simulink model "GlidePathControl_GlideSlopeAngle"  (R2018b)
settings: Solver=VariableStepAuto  StartTime=0.0  StopTime=30  RelTol=1e-3
libraries: simulink x1
settings Model: Creator=cdjsd  LastModifiedBy=cdjsd

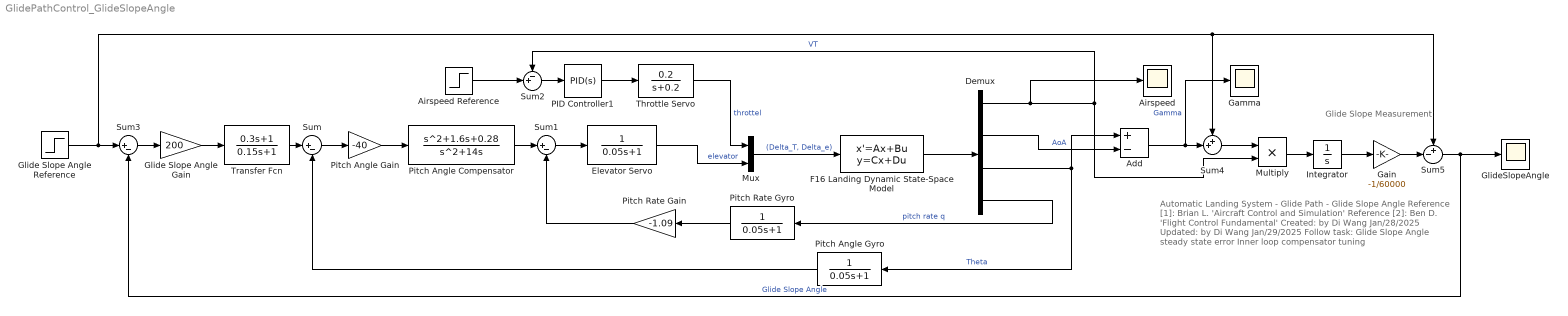
== system GlidePathControl_GlideSlopeAngle ==
  note: Glide Slope
      | Measurement
  note: Automatic Landing System - Glide Path - Glide Slope Angle
      | Reference [1]: Brian L. 'Aircraft Control and Simulation'
      | Reference [2]: Ben D. 'Flight Control Fundamental'
      | Created: by Di Wang Jan/28/2025
      | Updated: by Di Wang Jan/29/2025
      | Follow task: Glide Slope Angle steady state error
      | Inner loop compensator tuning
  Add : Sum  Inputs=+-
  Airspeed : Scope
  Airspeed Reference : Step  After=250  SampleTime=0
  Demux : Demux
  Elevator Servo : TransferFcn  Denominator=[0.05 1]
  F16 Landing Dynamic State-Space Model : StateSpace  A=|  B=[10.1 0; -1.5446e-4 0; 0 0; 0.024656 -0.01077]  C=[1 0 0 0; 0 57.296 0 0; 0 0 57.296 0; 0 0 0 57.296]  D=zeros(4,2)  InitialCondition=0
      | [-0.03858 18.984 -32.139 0;
      |      -0.001028 -0.63253 0.0056129 1;
      |      0 0 0 1;
      |      7.8601e-5 -0.75905 -0.00079341 -0.5183]
  Gain : Gain  Gain=-1/60000
  Gamma : Scope
  Glide Slope Angle Gain : Gain  Gain=200
  Glide Slope Angle Reference : Step  After=3  SampleTime=0
  GlideSlopeAngle : Scope
  Integrator : Integrator
  Multiply : Product
  Mux : Mux  Inputs=2
  PID Controller1 : simulink/Continuous/PID Controller  Controller=PID  Form=Parallel  TimeDomain=Continuous-time  SampleTime=-1  IntegratorMethod=Forward Euler  FilterMethod=Forward Euler  ControllerParametersSource=internal  P=0.231637684703423  I=0.0265486148062853  D=0.47251104710243  UseFilter=on  N=5.77992210933298  TunerSelectOption=Transfer Function Based (PID Tuner App)  InitialConditionSource=internal  InitialConditionForIntegrator=0  InitialConditionForFilter=0  DifferentiatorICPrevScaledInput=0  ExternalReset=none  TrackingMode=off  Kt=1  LimitOutput=off  UpperSaturationLimit=inf  LowerSaturationLimit=-inf  LinearizeAsGain=on  AntiWindupMode=none  Kb=1  POutMin=[]  POutMax=[]  IOutMin=[]  IOutMax=[]  DOutMin=[]  DOutMax=[]  NOutMin=[]  NOutMax=[]  SumOutMin=[]  SumOutMax=[]  SaturationOutMin=[]  SaturationOutMax=[]  PParamMin=[]  PParamMax=[]  IParamMin=[]  IParamMax=[]  DParamMin=[]  DParamMax=[]  NParamMin=[]  NParamMax=[]  KbParamMin=[]  KbParamMax=[]  KtParamMin=[]  KtParamMax=[]  KbOutMin=[]  KbOutMax=[]  KtOutMin=[]  KtOutMax=[]  IntegratorOutMin=[]  IntegratorOutMax=[]  FilterOutMin=[]  FilterOutMax=[]  SumI1OutMin=[]  SumI1OutMax=[]  SumI2OutMin=[]  SumI2OutMax=[]  SumI3OutMin=[]  SumI3OutMax=[]  SumI4OutMin=[]  SumI4OutMax=[]  SumDOutMin=[]  SumDOutMax=[]  DifferentiatorOutMin=[]  DifferentiatorOutMax=[]  FilterDiffOutCoefMin=[]  FilterDiffOutCoefMax=[]  ReciprocalOutMin=[]  ReciprocalOutMax=[]  SumDenOutMin=[]  SumDenOutMax=[]  SumNumOutMin=[]  SumNumOutMax=[]  DivideOutMin=[]  DivideOutMax=[]  IntegratorContinuousStateAttributes=''  IntegratorStateMustResolveToSignalObject=off  IntegratorRTWStateStorageClass=Auto  FilterContinuousStateAttributes=''  FilterStateMustResolveToSignalObject=off  FilterRTWStateStorageClass=Auto  ParallelPVariant=InternalParameters  IdealPVariant=Disabled  IVariant=InternalParameters  DVariant=InternalParameters  IntegratorVariant=Continuous  SatVariant=Disabled  AWVariant=Passthrough  PCopyVariant=Disabled  TRVariant=Disabled  FdbkBlocksVariant=Forward  IdealPFdbkVariant=Disabled  SatFdbkVariant=Disabled  DerivativeFilterVariant=ContFilter  NVariant=InternalParameters  NCopyVariant=Disabled  FilterICVariant=InternalICsFilter  IntegratorICVariant=InternalICs  ExternalResetVariant=Disabled  TRSumVariant=Passthrough  SumFdbkVariant=Disabled  SumVariant=Sum_PID
  Pitch Angle Compensator : TransferFcn  Numerator=[1 1.6 0.28]  Denominator=[1 14 0]
  Pitch Angle Gain : Gain  Gain=-40
  Pitch Angle Gyro : TransferFcn  Denominator=[0.05 1]
  Pitch Rate Gain : Gain  Gain=-1.09
  Pitch Rate Gyro : TransferFcn  Denominator=[0.05 1]
  Sum : Sum  Inputs=|+-
  Sum1 : Sum  Inputs=|+-
  Sum2 : Sum  Inputs=-+|
  Sum3 : Sum  Inputs=|+-
  Sum4 : Sum  Inputs=++|
  Sum5 : Sum  Inputs=+-|
  Throttle Servo : TransferFcn  Numerator=[0.2]  Denominator=[1 0.2]
  Transfer Fcn : TransferFcn  Numerator=[0.3 1]  Denominator=[0.15 1]
  wires:
  Mux/1 -> F16 Landing Dynamic State-Space Model/1  "(Delta_T, Delta_e)"
  Sum/1 -> Pitch Angle Gain/1
  F16 Landing Dynamic State-Space Model/1 -> Demux/1
  Demux/1 -> Airspeed/1, Multiply/2, Sum2/1  "VT"
  Demux/3 -> Add/1, Pitch Angle Gyro/1  "Theta"
  Demux/4 -> Pitch Rate Gyro/1  "pitch rate q"
  Elevator Servo/1 -> Mux/2  "elevator"
  Pitch Rate Gain/1 -> Sum1/2
  Sum1/1 -> Elevator Servo/1
  Pitch Rate Gyro/1 -> Pitch Rate Gain/1
  Pitch Angle Gyro/1 -> Sum/2
  Sum2/1 -> PID Controller1/1
  PID Controller1/1 -> Throttle Servo/1
  Throttle Servo/1 -> Mux/1  "throttel"
  Demux/2 -> Add/2  "AoA"
  Add/1 -> Gamma/1, Sum4/2  "Gamma"
  Sum4/1 -> Multiply/1
  Multiply/1 -> Integrator/1
  Integrator/1 -> Gain/1
  Gain/1 -> Sum5/2
  Sum5/1 -> Sum3/2, GlideSlopeAngle/1  "Glide Slope Angle"
  Airspeed Reference/1 -> Sum2/2
  Glide Slope Angle Reference/1 -> Sum3/1, Sum5/1, Sum4/1
  Sum3/1 -> Glide Slope Angle Gain/1
  Pitch Angle Gain/1 -> Pitch Angle Compensator/1
  Pitch Angle Compensator/1 -> Sum1/1
  Transfer Fcn/1 -> Sum/1
  Glide Slope Angle Gain/1 -> Transfer Fcn/1
